simulink model "High_pass"  (R2018a)
settings: Solver=VariableStepAuto  StartTime=0.0  StopTime=1.0  RelTol=1e-3
libraries: dsparch4 x1
settings Model: Creator=AlexZ  LastModifiedBy=AlexZ

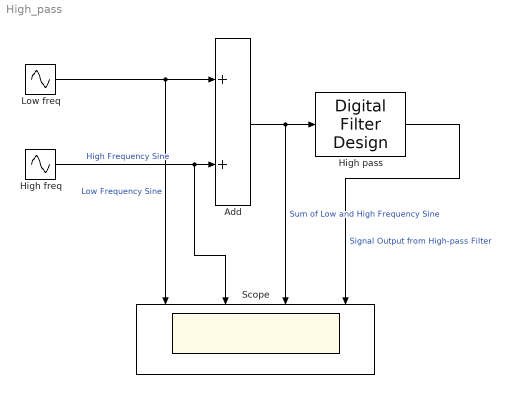
== system High_pass ==
  Add : Sum
  "High freq " : Sin  Frequency=2*pi*50  SampleTime=0.0001
  "High pass " : dsparch4/Digital Filter Design  mwdsp_browser_bugfix_var=off
  "Low freq " : Sin  Frequency=2*pi*10  SampleTime=0.0001
  Scope : Scope  NumInputPorts=4
  wires:
  "Low freq "/1 -> Add/1, Scope/1  "Low Frequency Sine"
  "High pass "/1 -> Scope/4  "Signal Output from High-pass Filter"
  "High freq "/1 -> Scope/2, Add/2  "High Frequency Sine"
  Add/1 -> "High pass "/1, Scope/3  "Sum of Low and High Frequency Sine"
